simulink model "simIC"  (R2023b)
settings: Solver=VariableStepAuto  StartTime=0.0  StopTime=100.0  RelTol=1e-3
values from neighbouring files (symbols this model uses):
  beta = .1    (= 0.1)    [runIC.m]
  D_d = eye(6)*3    [runIC.m]
  dragcoeff = [C_d_1, C_d_4, C_d_C, C_d_L, beta, gamma]    [runIC.m]
  G_d = eye(6)*0.5    [runIC.m]
  gamma = .1    (= 0.1)    [runIC.m]
  K_D = blkdiag(eye(3),eye(3),eye(9))*500    [runIC.m]
  K_DI = diag([0.5 0.5 0.5 0.1 0.1 0.1])*2    [runIC.m]
  K_II = diag([0.2 0.2 0.2 0.15 0.15 0.15]*20)    [runIC.m]
  K_P = blkdiag(eye(3),eye(3),eye(9)*30)    [runIC.m]
  K_SI = diag([1 1 1 0.2 0.2 0.2])*30    [runIC.m]
  Lambda = blkdiag(eye(3)*40,eye(3)*40,eye(9)*40)    [runIC.m]
  M_d = eye(6)*4    [runIC.m]
  pos_init = [-0.02 (2*0.77*cos(pi/4)+1) 0]    [runIC.m]
  quat_init = eul2quat([0 0 pi],'XYZ')    [runIC.m]
  theta_init = [0 pi/4 0 pi/4 pi/4 0 pi/4 0 0]    [runIC.m]
  x_init = [pos_init quat_init theta_init zeta_init]'    [runIC.m]
undefined symbols (not defined in the file or in its folder): dt_MPC, pp, snake
libraries: dspindex x4, cstblocks x3
settings Model: Creator=sarava  LastModifiedBy=asker
settings SolverCC: AlgebraicLoopSolver=TrustRegion
settings DataIOCC: ReturnWorkspaceOutputs=off
settings DebuggingCC: UnconnectedInputMsg=warning  UnconnectedOutputMsg=warning  UnconnectedLineMsg=warning  ArithmeticOperatorsInVariantConditions=warning
settings ModelReferenceCC: EnableRefExpFcnMdlSchedulingChecks=on
settings SFSimCC: SimUseLocalCustomCode=off  CustomCodeUndefinedFunction=UseInterfaceOnly
settings RTWCC: RTWUseLocalCustomCode=off

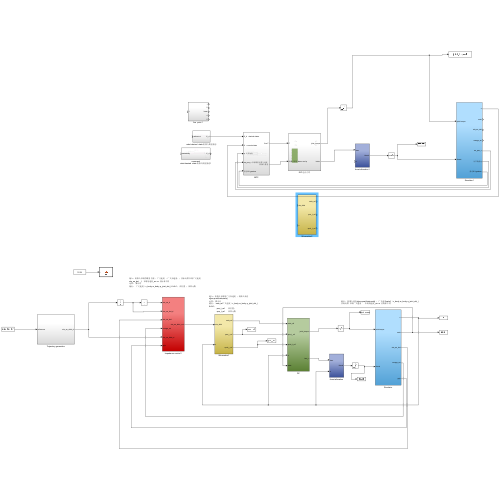
[thumbnail: Simulink's stored preview of the top-level diagram]
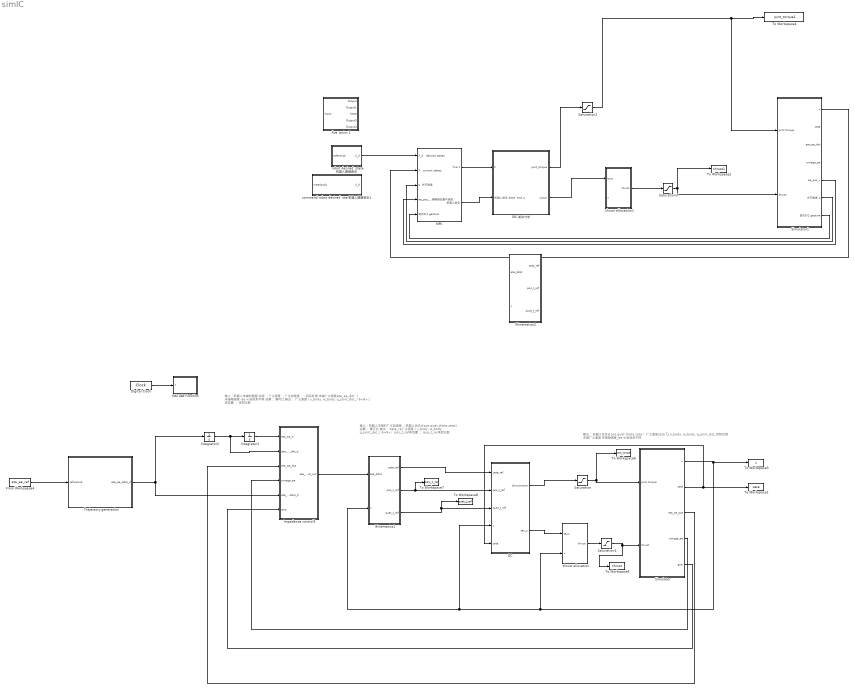
== system simIC ==
  note: 输入：机器人末端的广义加速度  ；机器人状态x[pos,quat,theta,zeta]
      | 运算： 雅可比
      | 输出：  zeta_ref广义速度（v_body, w_body, q_joint_dot_) 6+8+1；
      | 		pos_t_ref  	体位置 ；
      | 		qua_t_ref 	体四元数
  note: 输入：机器人末端的期望 位姿 ，广义速度  ，广义加速度，；实际反馈 末端广义速度eta_ee_dot   _I   末端角速度_ee  w  坐标系不同
      | 运算： 雅可比
      | 输出：  广义速度（v_body, w_body, q_joint_dot_) 6+8+1； 体位置 ； 体四元数
  note: 输出： 机器人状态x[pos,quat,theta,zeta]  ； 广义速度zeta ζ（v_body, w_body, q_joint_dot_)
      | 实际反馈  末端广义速度       末端角速度_ee  w  坐标系不同
  DC : Subsystem
  Digital Clock : DigitalClock
  From Workspace4 : FromWorkspace  VariableName=eta_ee_ref
  IDC 逆动力学 : Subsystem
  IKinematics1 : Subsystem
  IKinematics2 : Subsystem
  Impedance control1 : Subsystem
  Integrator1 : Integrator
  Integrator2 : Integrator
  MATLAB Function : MATLAB Function  TreatAsAtomicUnit=on
  MPC : Subsystem
  Saturation : Saturate  UpperLimit=8  LowerLimit=-2  ZeroCross=off
  Saturation1 : Saturate  UpperLimit=5  LowerLimit=-5  ZeroCross=off
  Saturation2 : Saturate  UpperLimit=8  LowerLimit=-2  ZeroCross=off
  Saturation3 : Saturate  UpperLimit=5  LowerLimit=-5  ZeroCross=off
  Simulator : Subsystem
  Simulator1 : Subsystem
  To Workspace1 : ToWorkspace  VariableName=zeta  SaveFormat=Timeseries  SampleTime=-1
  To Workspace2 : ToWorkspace  VariableName=thrust1  SaveFormat=Timeseries  SampleTime=-1
  To Workspace3 : ToWorkspace  VariableName=x  SaveFormat=Timeseries  SampleTime=-1
  To Workspace4 : ToWorkspace  VariableName=joint_torque1  SaveFormat=Timeseries  SampleTime=-1
  To Workspace5 : ToWorkspace  VariableName=thrust  SaveFormat=Timeseries  SampleTime=-1
  To Workspace6 : ToWorkspace  VariableName=joint_torque  SaveFormat=Timeseries  SampleTime=-1
  To Workspace7 : ToWorkspace  VariableName=pos_t_ref  SaveFormat=Timeseries  SampleTime=-1
  To Workspace8 : ToWorkspace  VariableName=quat_t_ref  SaveFormat=Timeseries  SampleTime=-1
  "Trajectory generation " : Subsystem
  command robot desired  state 机器人期望姿态1 : Subsystem
  five  point 1 : Subsystem
  robot desired  state 机器人期望姿态 : Subsystem
  thrust allocation : Subsystem
  thrust allocation1 : Subsystem
  wires:
  Digital Clock/1 -> MATLAB Function/1(t)
  thrust allocation/1(thrust) -> Saturation1/1
  Simulator/2(zeta) -> To Workspace1/1, DC/5("zeta ")
  Simulator/1(x) -> To Workspace3/1, DC/4(x), IKinematics1/2(x), thrust allocation/2("x ")
  IKinematics1/2(pos_t_ref) -> DC/2(pos_t_ref), To Workspace7/1
  IKinematics1/1(zeta_ref) -> DC/1(zeta_ref)
  IKinematics1/3(quat_t_ref) -> To Workspace8/1, DC/3(quat_t_ref)
  From Workspace4/1 -> "Trajectory generation "/1(reference)
  Integrator2/1 -> Impedance control1/2(eta_ee_dot_d), Integrator1/1
  "Trajectory generation "/1(eta_ee_ddot_d) -> Integrator2/1, Impedance control1/5(eta_ee_ddot_d)
  Simulator/3(eta_ee_dot) -> Impedance control1/3(eta_ee_dot)
  Simulator/4(omega_ee) -> Impedance control1/4(omega_ee)
  Integrator1/1 -> Impedance control1/1(eta_ee_d)
  Impedance control1/1(eta_ee_ddot_out) -> IKinematics1/1(eta_ddot)
  Simulator/5(grip) -> Impedance control1/6(grip)
  Saturation/1 -> To Workspace6/1, Simulator/1(joint torque)
  Saturation1/1 -> To Workspace5/1, Simulator/2(thrust)
  DC/1(joint_torque) -> Saturation/1
  DC/2(tau_c) -> thrust allocation/1("tauc ")
  Saturation2/1 -> To Workspace4/1, Simulator1/1(joint torque)
  IDC 逆动力学/1(joint_torque) -> Saturation2/1
  Saturation3/1 -> To Workspace2/1, Simulator1/2(thrust)
  thrust allocation1/1(thrust) -> Saturation3/1
  IDC 逆动力学/2("turtor ") -> thrust allocation1/1("tauc ")
  MPC/1(five F) -> IDC 逆动力学/1(F)
  MPC/2("机器人姿态 ") -> IDC 逆动力学/2(机器人姿态 base  and q)
  Simulator1/1(x) -> MPC/2(X   current states)
  Simulator1/6(关节角度 q) -> MPC/3(q  关节角度)
  Simulator1/5(ee_pos_v) -> MPC/4(ee_pos_v 末端期望位置与速度)
  robot desired  state 机器人期望姿态/1(X_d) -> MPC/1(X_d   desired states)
  Simulator1/7(姿态0/1 gesture) -> MPC/5(姿态0/1 gesture)

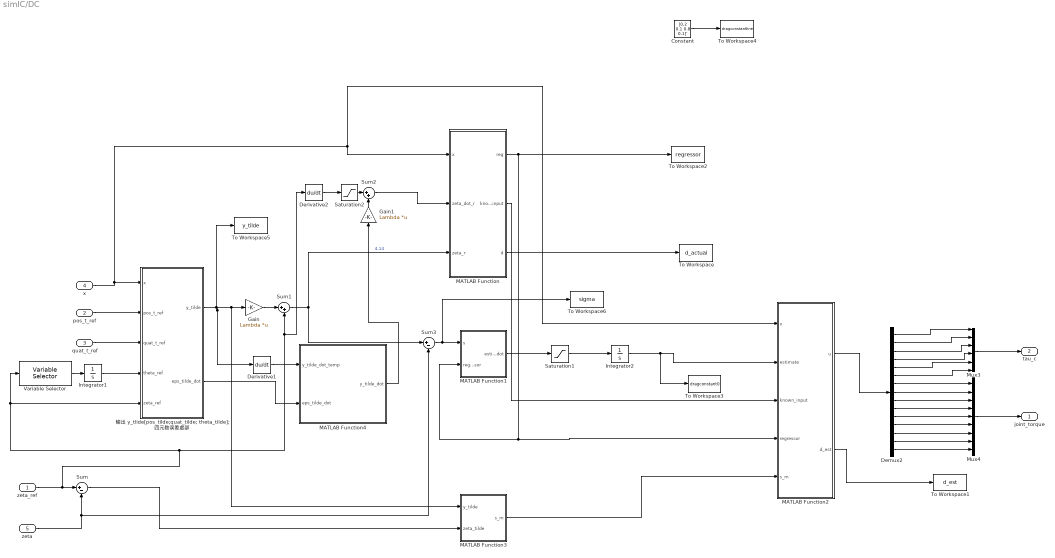
== system simIC/DC ==
  zeta_ref : Inport
  pos_t_ref : Inport  Port=2
  quat_t_ref : Inport  Port=3
  x : Inport  Port=4
  "zeta " : Inport  Port=5
  Constant : Constant  Value=[0.2 0.1 0.8 0.1]'
  Demux2 : Demux  Outputs=15
  Derivative1 : Derivative  CoefficientInTFapproximation=10
  Derivative2 : Derivative  CoefficientInTFapproximation=10
  Gain : Gain  Gain=Lambda  Multiplication=Matrix(K*u) (u vector)
  Gain1 : Gain  Gain=Lambda  Multiplication=Matrix(K*u) (u vector)
  Integrator1 : Integrator  InitialCondition=theta_init
  Integrator2 : Integrator  InitialCondition=[0 0 0 0]'
  MATLAB Function : MATLAB Function  TreatAsAtomicUnit=on
  MATLAB Function1 : MATLAB Function  TreatAsAtomicUnit=on
  MATLAB Function2 : MATLAB Function  TreatAsAtomicUnit=on
  MATLAB Function3 : MATLAB Function  TreatAsAtomicUnit=on
  MATLAB Function4 : MATLAB Function  TreatAsAtomicUnit=on
  Mux3 : Mux  Inputs=6
  Mux4 : Mux  Inputs=9
  Saturation1 : Saturate  UpperLimit=50  LowerLimit=-50  ZeroCross=off
  Saturation2 : Saturate  UpperLimit=20  LowerLimit=-20  ZeroCross=off
  Sum : Sum  Inputs=|+-
  Sum1 : Sum  Inputs=|++
  Sum2 : Sum  Inputs=|++
  Sum3 : Sum  Inputs=|+-
  To Workspace : ToWorkspace  VariableName=d_actual  SaveFormat=Timeseries  SampleTime=-1
  To Workspace1 : ToWorkspace  VariableName=d_est  SaveFormat=Timeseries  SampleTime=-1
  To Workspace2 : ToWorkspace  VariableName=regressor  SaveFormat=Timeseries  SampleTime=-1
  To Workspace3 : ToWorkspace  VariableName=dragconstant0  SaveFormat=Timeseries  SampleTime=-1
  To Workspace4 : ToWorkspace  VariableName=dragconstantline  SaveFormat=Timeseries  SampleTime=-1
  To Workspace5 : ToWorkspace  VariableName=y_tilde  SaveFormat=Timeseries  SampleTime=-1
  To Workspace6 : ToWorkspace  VariableName=sigma  SaveFormat=Timeseries  SampleTime=-1
  Variable Selector : dspindex/Variable Selector  NumInputs=1  rowsOrCols=Rows  IdxMode=Fixed  Elements=7:15  ZerOneIdxMode=One-based  errmode=Clip Index  FillMode=on  FillValues=0
  输出 y_tlide[pos_tilde;quat_tilde; theta_tilde]; 四元数误差虚部 : MATLAB Function  TreatAsAtomicUnit=on
  joint_torque : Outport  VectorParamsAs1DForOutWhenUnconnected=off
  tau_c : Outport  Port=2  VectorParamsAs1DForOutWhenUnconnected=off
  wires:
  x/1 -> MATLAB Function/1(x), MATLAB Function2/1(x), 输出 y_tlide[pos_tilde;quat_tilde; theta_tilde]; 四元数误差虚部/1(x)
  pos_t_ref/1 -> 输出 y_tlide[pos_tilde;quat_tilde; theta_tilde]; 四元数误差虚部/2(pos_t_ref)
  quat_t_ref/1 -> 输出 y_tlide[pos_tilde;quat_tilde; theta_tilde]; 四元数误差虚部/3(quat_t_ref)
  zeta_ref/1 -> Derivative2/1, Sum1/2, Variable Selector/1, 输出 y_tlide[pos_tilde;quat_tilde; theta_tilde]; 四元数误差虚部/5(zeta_ref), Sum/1
  "zeta "/1 -> Sum3/2, Sum/2
  Integrator1/1 -> 输出 y_tlide[pos_tilde;quat_tilde; theta_tilde]; 四元数误差虚部/4(theta_ref)
  输出 y_tlide[pos_tilde;quat_tilde; theta_tilde]; 四元数误差虚部/1(y_tilde) -> MATLAB Function3/1(y_tilde), Gain/1, Derivative1/1, To Workspace5/1
  Gain/1 -> Sum1/1
  Sum1/1 -> Sum3/1, MATLAB Function/3(zeta_r)  "4.14"
  Saturation1/1 -> Integrator2/1
  MATLAB Function1/1(estimate_dot) -> Saturation1/1
  MATLAB Function3/1(s_m) -> MATLAB Function2/5(s_m)
  MATLAB Function2/1(u) -> Demux2/1
  Demux2/14 -> Mux4/8
  Demux2/4 -> Mux3/4
  Demux2/5 -> Mux3/5
  Demux2/12 -> Mux4/6
  Demux2/2 -> Mux3/2
  Demux2/9 -> Mux4/3
  Demux2/3 -> Mux3/3
  Demux2/13 -> Mux4/7
  Demux2/8 -> Mux4/2
  Demux2/6 -> Mux3/6
  Demux2/10 -> Mux4/4
  Demux2/7 -> Mux4/1
  Demux2/11 -> Mux4/5
  Demux2/1 -> Mux3/1
  Mux4/1 -> joint_torque/1
  Mux3/1 -> tau_c/1
  Variable Selector/1 -> Integrator1/1
  Integrator2/1 -> To Workspace3/1, MATLAB Function2/2(estimate)
  MATLAB Function/2(known_input) -> MATLAB Function2/3(known_input)
  MATLAB Function/1(reg) -> To Workspace2/1, MATLAB Function1/2(regressor), MATLAB Function2/4(regressor)
  输出 y_tlide[pos_tilde;quat_tilde; theta_tilde]; 四元数误差虚部/2(eps_tilde_dot) -> MATLAB Function4/2(eps_tilde_dot)
  Derivative1/1 -> MATLAB Function4/1(y_tilde_dot_temp)
  MATLAB Function4/1(y_tilde_dot) -> Gain1/1
  Derivative2/1 -> Saturation2/1
  Saturation2/1 -> Sum2/1
  Gain1/1 -> Sum2/2
  Sum3/1 -> To Workspace6/1, MATLAB Function1/1(s)
  Sum2/1 -> MATLAB Function/2(zeta_dot_r)
  Sum/1 -> MATLAB Function3/2(zeta_tilde)
  MATLAB Function/3(d) -> To Workspace/1
  MATLAB Function2/2(d_est) -> To Workspace1/1
  Constant/1 -> To Workspace4/1
  Demux2/15 -> Mux4/9

== system simIC/IDC 逆动力学 ==
  F : Inport
  机器人姿态 base  and q : Inport  Port=2
  DC : Subsystem
  joint_torque : Outport
  "turtor " : Outport  Port=2

== system simIC/IKinematics1 ==
  eta_ddot : Inport
  x : Inport  Port=2
  Integrator3 : Integrator
  Integrator5 : Integrator  InitialCondition=[pos_init quat_init]'
  MATLAB Function1 : MATLAB Function  TreatAsAtomicUnit=on
  zeta_ref : Outport  VectorParamsAs1DForOutWhenUnconnected=off
  pos_t_ref : Outport  Port=2  VectorParamsAs1DForOutWhenUnconnected=off
  quat_t_ref : Outport  Port=3  VectorParamsAs1DForOutWhenUnconnected=off
  wires:
  x/1 -> MATLAB Function1/2(x)
  MATLAB Function1/1(zeta_ref) -> zeta_ref/1
  MATLAB Function1/2(pos_t_ref) -> pos_t_ref/1
  eta_ddot/1 -> Integrator3/1
  Integrator3/1 -> MATLAB Function1/1(eta_ee_d_dot)
  MATLAB Function1/3(eta_t_dot_quat_ref) -> Integrator5/1
  Integrator5/1 -> MATLAB Function1/3(eta_t_ref)
  MATLAB Function1/4(quatt_ref) -> quat_t_ref/1

== system simIC/IKinematics2 ==
  eta_ddot : Inport
  x : Inport  Port=2
  Integrator3 : Integrator
  Integrator5 : Integrator  InitialCondition=[pos_init quat_init]'
  MATLAB Function1 : MATLAB Function  TreatAsAtomicUnit=on
  zeta_ref : Outport  VectorParamsAs1DForOutWhenUnconnected=off
  pos_t_ref : Outport  Port=2  VectorParamsAs1DForOutWhenUnconnected=off
  quat_t_ref : Outport  Port=3  VectorParamsAs1DForOutWhenUnconnected=off
  wires:
  x/1 -> MATLAB Function1/3(x)
  MATLAB Function1/1(zeta_ref) -> zeta_ref/1
  MATLAB Function1/2(pos_t_ref) -> pos_t_ref/1
  eta_ddot/1 -> Integrator3/1
  Integrator3/1 -> MATLAB Function1/1(eta_zuo_d_dot)
  MATLAB Function1/3(eta_t_dot_quat_ref) -> Integrator5/1
  Integrator5/1 -> MATLAB Function1/4(eta_t_ref)
  MATLAB Function1/4(quatt_ref) -> quat_t_ref/1

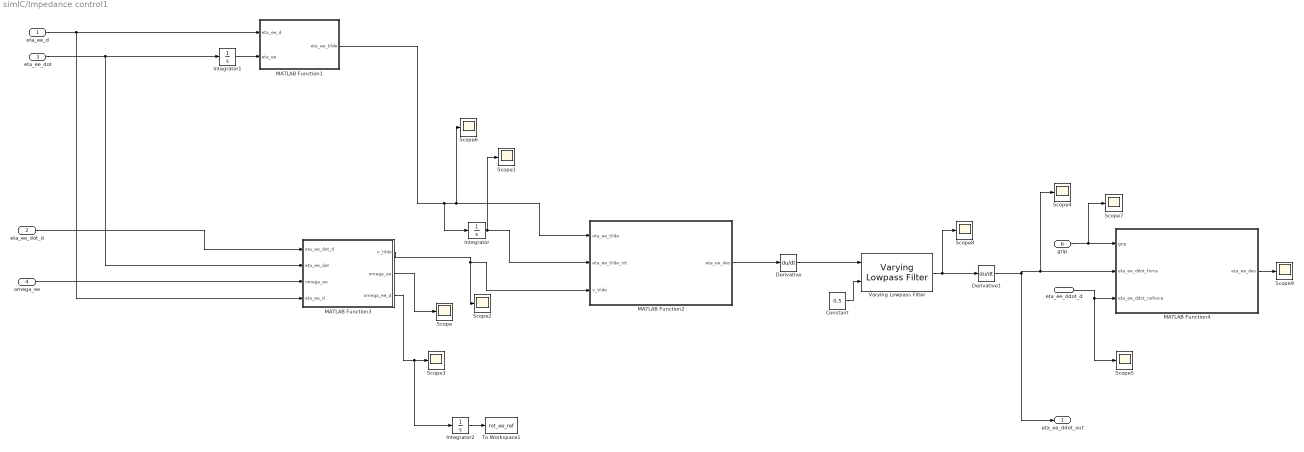
== system simIC/Impedance control1 ==
  eta_ee_d : Inport
  eta_ee_dot_d : Inport  Port=2
  eta_ee_dot : Inport  Port=3
  omega_ee : Inport  Port=4
  eta_ee_ddot_d : Inport  Port=5
  grip : Inport  Port=6
  Constant : Constant  Value=0.5
  Derivative : Derivative
  Derivative1 : Derivative
  Integrator : Integrator
  Integrator1 : Integrator
  Integrator2 : Integrator
  MATLAB Function1 : MATLAB Function  TreatAsAtomicUnit=on
  MATLAB Function2 : MATLAB Function  TreatAsAtomicUnit=on
  MATLAB Function3 : MATLAB Function  TreatAsAtomicUnit=on
  MATLAB Function4 : MATLAB Function  TreatAsAtomicUnit=on
  Scope{,1..9} (10 alike) : Scope
  To Workspace1 : ToWorkspace  VariableName=rot_ee_ref  SaveFormat=Timeseries  SampleTime=-1
  Varying Lowpass Filter : cstblocks/Linear Parameter Varying/Varying Lowpass Filter  N=1
  eta_ee_ddot_out : Outport  VectorParamsAs1DForOutWhenUnconnected=off
  wires:
  eta_ee_d/1 -> MATLAB Function3/4(eta_ee_d), MATLAB Function1/1(eta_ee_d)
  eta_ee_dot_d/1 -> MATLAB Function3/1(eta_ee_dot_d)
  eta_ee_dot/1 -> Integrator1/1, MATLAB Function3/2(eta_ee_dot)
  omega_ee/1 -> MATLAB Function3/3("omega_ee ")
  MATLAB Function3/1(v_tilde) -> MATLAB Function2/3(v_tilde), Scope2/1
  MATLAB Function1/1(eta_ee_tilde) -> Integrator/1, Scope6/1, MATLAB Function2/1(eta_ee_tilde)
  Integrator/1 -> Scope1/1, MATLAB Function2/2(eta_ee_tilde_int)
  MATLAB Function3/2(omega_ee) -> Scope/1
  MATLAB Function2/1(eta_ee_des) -> Derivative/1
  Integrator1/1 -> MATLAB Function1/2(eta_ee)
  MATLAB Function3/3(omega_ee_d) -> Integrator2/1, Scope3/1
  Constant/1 -> Varying Lowpass Filter/2
  Derivative/1 -> Varying Lowpass Filter/1
  Varying Lowpass Filter/1 -> Derivative1/1, Scope8/1
  Integrator2/1 -> To Workspace1/1
  grip/1 -> Scope7/1, MATLAB Function4/1(grip)
  Derivative1/1 -> eta_ee_ddot_out/1, Scope4/1, MATLAB Function4/2(eta_ee_ddot_force)
  eta_ee_ddot_d/1 -> Scope5/1, MATLAB Function4/3(eta_ee_ddot_noforce)
  MATLAB Function4/1(eta_ee_des) -> Scope9/1

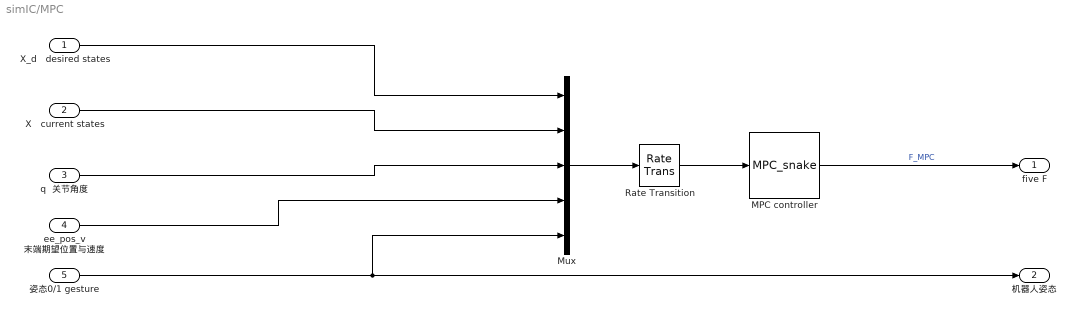
== system simIC/MPC ==
  X_d   desired states : Inport
  X   current states : Inport  Port=2
  q  关节角度 : Inport  Port=3
  ee_pos_v 末端期望位置与速度 : Inport  Port=4
  姿态0/1 gesture : Inport  Port=5
  MPC controller : MATLABFcn  MATLABFcn=MPC_snake  OutputDimensions=[12 1]  Output1D=off
  Mux : Mux  Inputs=5
  Rate Transition : RateTransition  OutPortSampleTime=dt_MPC/5
  five F : Outport
  "机器人姿态 " : Outport  Port=2
  wires:
  Mux/1 -> Rate Transition/1
  X_d   desired states/1 -> Mux/1
  Rate Transition/1 -> MPC controller/1
  X   current states/1 -> Mux/2
  q  关节角度/1 -> Mux/3
  ee_pos_v 末端期望位置与速度/1 -> Mux/4
  姿态0/1 gesture/1 -> Mux/5, "机器人姿态 "/1
  MPC controller/1 -> five F/1  "F_MPC"

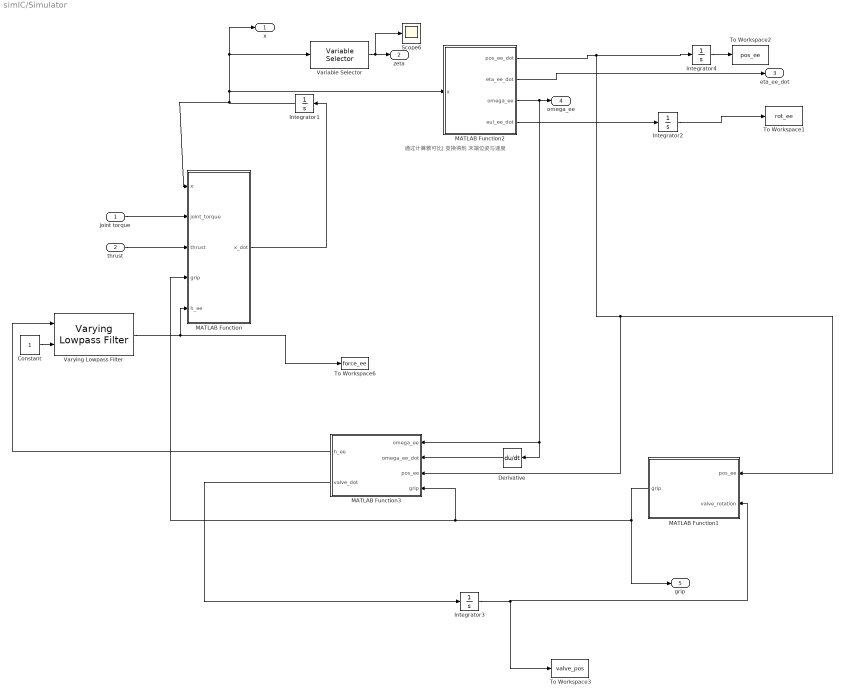
== system simIC/Simulator ==
  note: 通过计算雅可比J 变换得到 末端位姿与速度
  joint torque : Inport
  thrust : Inport  Port=2
  Constant : Constant
  Derivative : Derivative
  Integrator1 : Integrator  InitialCondition=x_init
  Integrator2 : Integrator
  Integrator3 : Integrator
  Integrator4 : Integrator
  MATLAB Function : MATLAB Function  TreatAsAtomicUnit=on
  MATLAB Function1 : MATLAB Function  TreatAsAtomicUnit=on
  MATLAB Function2 : MATLAB Function  TreatAsAtomicUnit=on
  MATLAB Function3 : MATLAB Function  TreatAsAtomicUnit=on
  Scope6 : Scope
  To Workspace1 : ToWorkspace  VariableName=rot_ee  SaveFormat=Timeseries  SampleTime=-1
  To Workspace2 : ToWorkspace  VariableName=pos_ee  SaveFormat=Timeseries  SampleTime=-1
  To Workspace3 : ToWorkspace  VariableName=valve_pos  SaveFormat=Timeseries  SampleTime=-1
  To Workspace6 : ToWorkspace  VariableName=force_ee  SaveFormat=Timeseries  SampleTime=-1
  Variable Selector : dspindex/Variable Selector  NumInputs=1  rowsOrCols=Rows  IdxMode=Fixed  Elements=17:31  ZerOneIdxMode=One-based  errmode=Clip Index  FillMode=on  FillValues=0
  Varying Lowpass Filter : cstblocks/Linear Parameter Varying/Varying Lowpass Filter  N=1
  x : Outport  VectorParamsAs1DForOutWhenUnconnected=off
  zeta : Outport  Port=2  VectorParamsAs1DForOutWhenUnconnected=off
  eta_ee_dot : Outport  Port=3  VectorParamsAs1DForOutWhenUnconnected=off
  omega_ee : Outport  Port=4  VectorParamsAs1DForOutWhenUnconnected=off
  grip : Outport  Port=5  VectorParamsAs1DForOutWhenUnconnected=off
  wires:
  joint torque/1 -> MATLAB Function/2(joint_torque)
  thrust/1 -> MATLAB Function/3(thrust)
  Variable Selector/1 -> Scope6/1, zeta/1
  MATLAB Function2/1(pos_ee_dot) -> Integrator4/1, MATLAB Function3/3(pos_ee), MATLAB Function1/1(pos_ee)
  MATLAB Function/1(x_dot) -> Integrator1/1
  Integrator1/1 -> Variable Selector/1, x/1, MATLAB Function2/1(x), MATLAB Function/1(x)
  MATLAB Function2/2(eta_ee_dot) -> eta_ee_dot/1
  MATLAB Function2/3(omega_ee) -> Derivative/1, MATLAB Function3/1(omega_ee), omega_ee/1
  Integrator2/1 -> To Workspace1/1
  MATLAB Function3/1(h_ee) -> Varying Lowpass Filter/1
  MATLAB Function1/1(grip) -> MATLAB Function3/4(grip), MATLAB Function/4(grip), grip/1
  MATLAB Function3/2(valve_dot) -> Integrator3/1
  Integrator3/1 -> MATLAB Function1/2(valve_rotation), To Workspace3/1
  Derivative/1 -> MATLAB Function3/2(omega_ee_dot)
  Varying Lowpass Filter/1 -> MATLAB Function/5(h_ee), To Workspace6/1
  Constant/1 -> Varying Lowpass Filter/2
  Integrator4/1 -> To Workspace2/1
  MATLAB Function2/4(eul_ee_dot) -> Integrator2/1

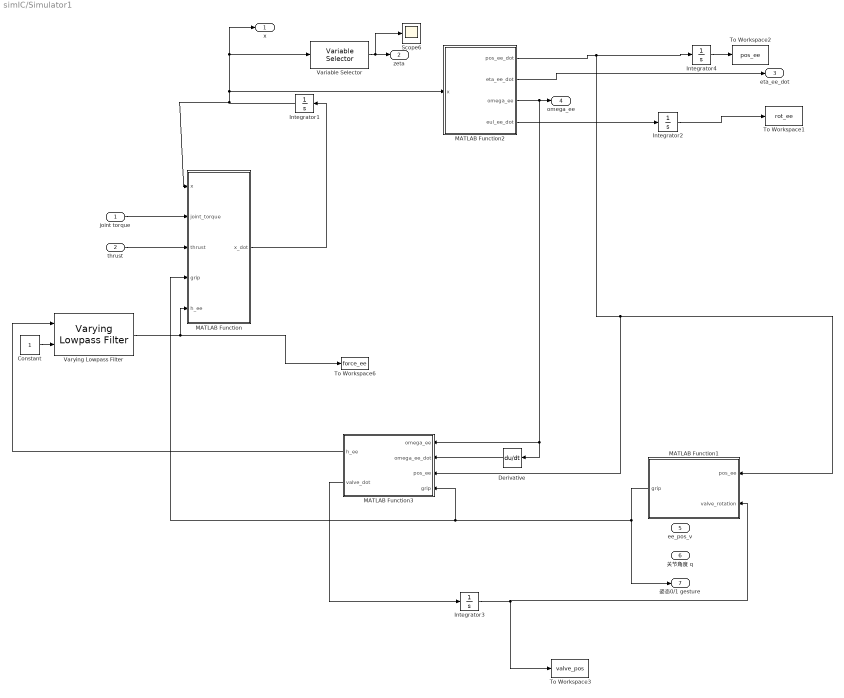
== system simIC/Simulator1 ==
  joint torque : Inport
  thrust : Inport  Port=2
  Constant : Constant
  Derivative : Derivative
  Integrator1 : Integrator  InitialCondition=x_init
  Integrator2 : Integrator
  Integrator3 : Integrator
  Integrator4 : Integrator
  MATLAB Function : MATLAB Function  TreatAsAtomicUnit=on
  MATLAB Function1 : MATLAB Function  TreatAsAtomicUnit=on
  MATLAB Function2 : MATLAB Function  TreatAsAtomicUnit=on
  MATLAB Function3 : MATLAB Function  TreatAsAtomicUnit=on
  Scope6 : Scope
  To Workspace1 : ToWorkspace  VariableName=rot_ee  SaveFormat=Timeseries  SampleTime=-1
  To Workspace2 : ToWorkspace  VariableName=pos_ee  SaveFormat=Timeseries  SampleTime=-1
  To Workspace3 : ToWorkspace  VariableName=valve_pos  SaveFormat=Timeseries  SampleTime=-1
  To Workspace6 : ToWorkspace  VariableName=force_ee  SaveFormat=Timeseries  SampleTime=-1
  Variable Selector : dspindex/Variable Selector  NumInputs=1  rowsOrCols=Rows  IdxMode=Fixed  Elements=17:31  ZerOneIdxMode=One-based  errmode=Clip Index  FillMode=on  FillValues=0
  Varying Lowpass Filter : cstblocks/Linear Parameter Varying/Varying Lowpass Filter  N=1
  x : Outport  VectorParamsAs1DForOutWhenUnconnected=off
  zeta : Outport  Port=2  VectorParamsAs1DForOutWhenUnconnected=off
  eta_ee_dot : Outport  Port=3  VectorParamsAs1DForOutWhenUnconnected=off
  omega_ee : Outport  Port=4  VectorParamsAs1DForOutWhenUnconnected=off
  ee_pos_v : Outport  Port=5
  关节角度 q : Outport  Port=6
  姿态0/1 gesture : Outport  Port=7  VectorParamsAs1DForOutWhenUnconnected=off
  wires:
  joint torque/1 -> MATLAB Function/2(joint_torque)
  thrust/1 -> MATLAB Function/3(thrust)
  Variable Selector/1 -> Scope6/1, zeta/1
  MATLAB Function2/1(pos_ee_dot) -> Integrator4/1, MATLAB Function3/3(pos_ee), MATLAB Function1/1(pos_ee)
  MATLAB Function/1(x_dot) -> Integrator1/1
  Integrator1/1 -> Variable Selector/1, x/1, MATLAB Function2/1(x), MATLAB Function/1(x)
  MATLAB Function2/2(eta_ee_dot) -> eta_ee_dot/1
  MATLAB Function2/3(omega_ee) -> Derivative/1, MATLAB Function3/1(omega_ee), omega_ee/1
  Integrator2/1 -> To Workspace1/1
  MATLAB Function3/1(h_ee) -> Varying Lowpass Filter/1
  MATLAB Function1/1(grip) -> MATLAB Function3/4(grip), MATLAB Function/4(grip), 姿态0/1 gesture/1
  MATLAB Function3/2(valve_dot) -> Integrator3/1
  Integrator3/1 -> MATLAB Function1/2(valve_rotation), To Workspace3/1
  Derivative/1 -> MATLAB Function3/2(omega_ee_dot)
  Varying Lowpass Filter/1 -> MATLAB Function/5(h_ee), To Workspace6/1
  Constant/1 -> Varying Lowpass Filter/2
  Integrator4/1 -> To Workspace2/1
  MATLAB Function2/4(eul_ee_dot) -> Integrator2/1

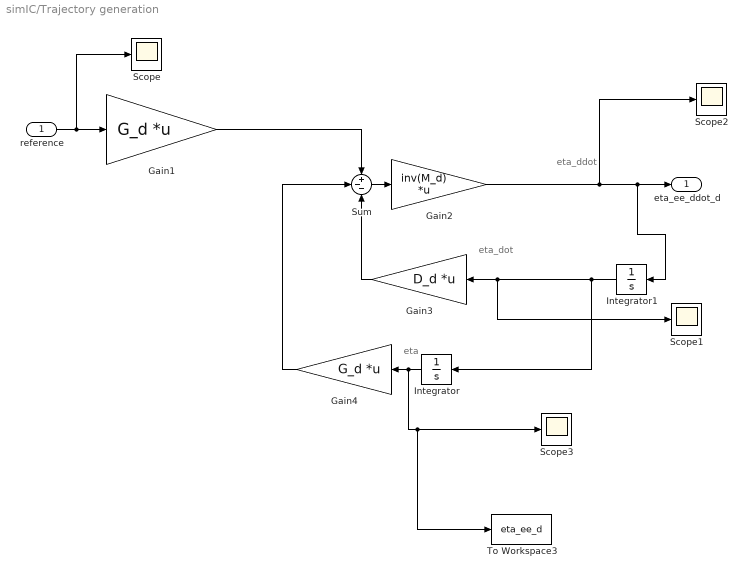
== system simIC/Trajectory generation  ==
  note: eta_dot
  note: eta
  note: eta_ddot
  reference : Inport
  Gain1 : Gain  Gain=G_d  Multiplication=Matrix(K*u) (u vector)
  Gain2 : Gain  Gain=inv(M_d)  Multiplication=Matrix(K*u) (u vector)
  Gain3 : Gain  Gain=D_d  Multiplication=Matrix(K*u) (u vector)
  Gain4 : Gain  Gain=G_d  Multiplication=Matrix(K*u) (u vector)
  Integrator : Integrator
  Integrator1 : Integrator
  Scope{,1..3} (4 alike) : Scope
  Sum : Sum  Inputs=+--
  To Workspace3 : ToWorkspace  VariableName=eta_ee_d  SaveFormat=Timeseries  SampleTime=-1
  eta_ee_ddot_d : Outport  VectorParamsAs1DForOutWhenUnconnected=off
  wires:
  Gain2/1 -> Scope2/1, eta_ee_ddot_d/1, Integrator1/1
  Gain1/1 -> Sum/1
  Sum/1 -> Gain2/1
  reference/1 -> Scope/1, Gain1/1
  Integrator1/1 -> Integrator/1, Scope1/1, Gain3/1
  Integrator/1 -> To Workspace3/1, Scope3/1, Gain4/1
  Gain3/1 -> Sum/3
  Gain4/1 -> Sum/2

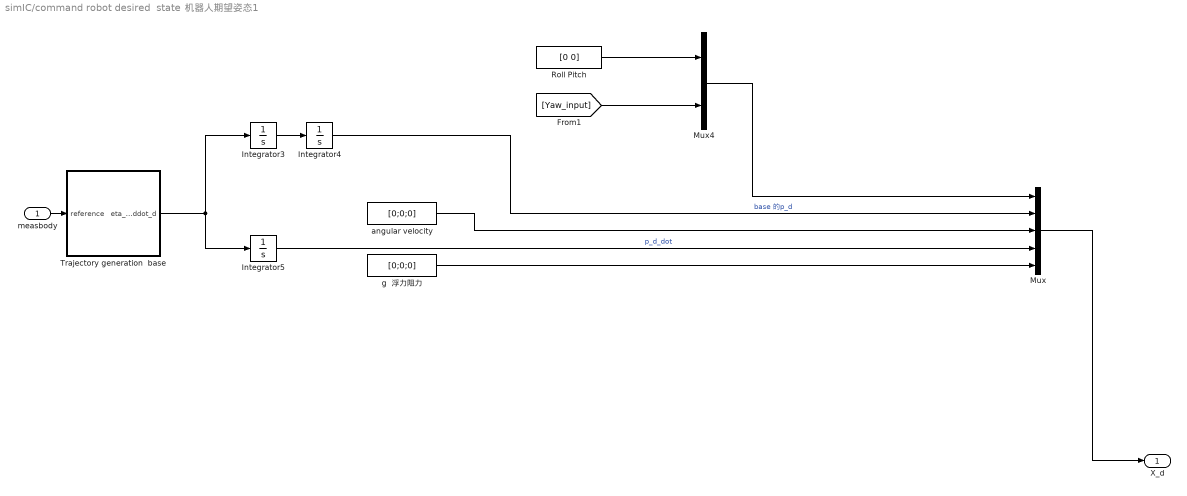
== system simIC/command robot desired  state 机器人期望姿态1 ==
  measbody : Inport
  Integrator3 : Integrator
  Integrator4 : Integrator
  Integrator5 : Integrator
  Mux : Mux  Inputs=5
  Mux4 : Mux  Inputs=2
  Roll Pitch : Constant  Value=[0 0]
  Trajectory generation  base : Subsystem
  angular velocity : Constant  Value=[0;0;0]
  g  浮力阻力 : Constant  Value=[0;0;0]
  X_d : Outport
  wires:
  Mux/1 -> X_d/1
  Mux4/1 -> Mux/1
  Integrator3/1 -> Integrator4/1
  [Yaw_input] -> Mux4/2
  g  浮力阻力/1 -> Mux/5
  Integrator5/1 -> Mux/4  "p_d_dot"
  Trajectory generation  base/1(eta_ee_ddot_d) -> Integrator3/1, Integrator5/1
  Roll Pitch/1 -> Mux4/1
  angular velocity/1 -> Mux/3
  measbody/1 -> Trajectory generation  base/1(reference)
  Integrator4/1 -> Mux/2  "base 的p_d"

== system simIC/five  point 1 ==
  Input : Inport
  Output : Outport
  Output1 : Outport  Port=2
  base : Outport  Port=3
  Output3 : Outport  Port=4
  Output4 : Outport  Port=5
  wires:
  Input/1 -> base/1

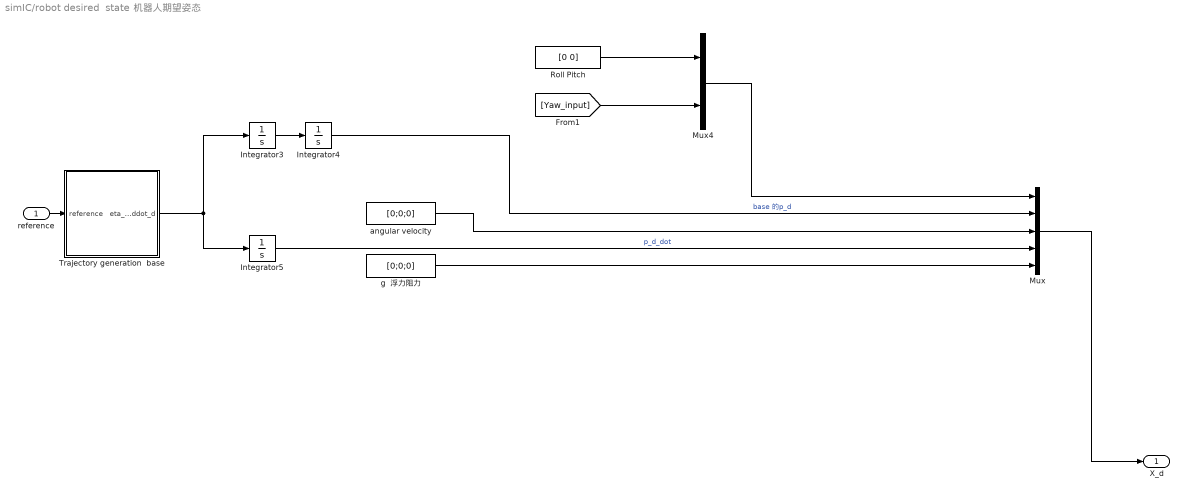
== system simIC/robot desired  state 机器人期望姿态 ==
  reference : Inport
  Integrator3 : Integrator
  Integrator4 : Integrator
  Integrator5 : Integrator
  Mux : Mux  Inputs=5
  Mux4 : Mux  Inputs=2
  Roll Pitch : Constant  Value=[0 0]
  Trajectory generation  base : Subsystem
  angular velocity : Constant  Value=[0;0;0]
  g  浮力阻力 : Constant  Value=[0;0;0]
  X_d : Outport
  wires:
  Mux/1 -> X_d/1
  Mux4/1 -> Mux/1
  Integrator3/1 -> Integrator4/1
  [Yaw_input] -> Mux4/2
  g  浮力阻力/1 -> Mux/5
  Integrator5/1 -> Mux/4  "p_d_dot"
  Trajectory generation  base/1(eta_ee_ddot_d) -> Integrator3/1, Integrator5/1
  Roll Pitch/1 -> Mux4/1
  angular velocity/1 -> Mux/3
  reference/1 -> Trajectory generation  base/1(reference)
  Integrator4/1 -> Mux/2  "base 的p_d"

== system simIC/thrust allocation ==
  "tauc " : Inport
  "x " : Inport  Port=2
  MATLAB Function : MATLAB Function  TreatAsAtomicUnit=on
  Product : Product  Multiplication=Matrix(*)
  thrust : Outport  VectorParamsAs1DForOutWhenUnconnected=off
  wires:
  "x "/1 -> MATLAB Function/1(x)
  MATLAB Function/1(TCM) -> Product/1
  "tauc "/1 -> Product/2
  Product/1 -> thrust/1

== system simIC/thrust allocation1 ==
  "tauc " : Inport
  "x " : Inport  Port=2
  MATLAB Function : MATLAB Function  TreatAsAtomicUnit=on
  Product : Product  Multiplication=Matrix(*)
  thrust : Outport  VectorParamsAs1DForOutWhenUnconnected=off
  wires:
  "x "/1 -> MATLAB Function/1(x)
  MATLAB Function/1(TCM) -> Product/1
  "tauc "/1 -> Product/2
  Product/1 -> thrust/1

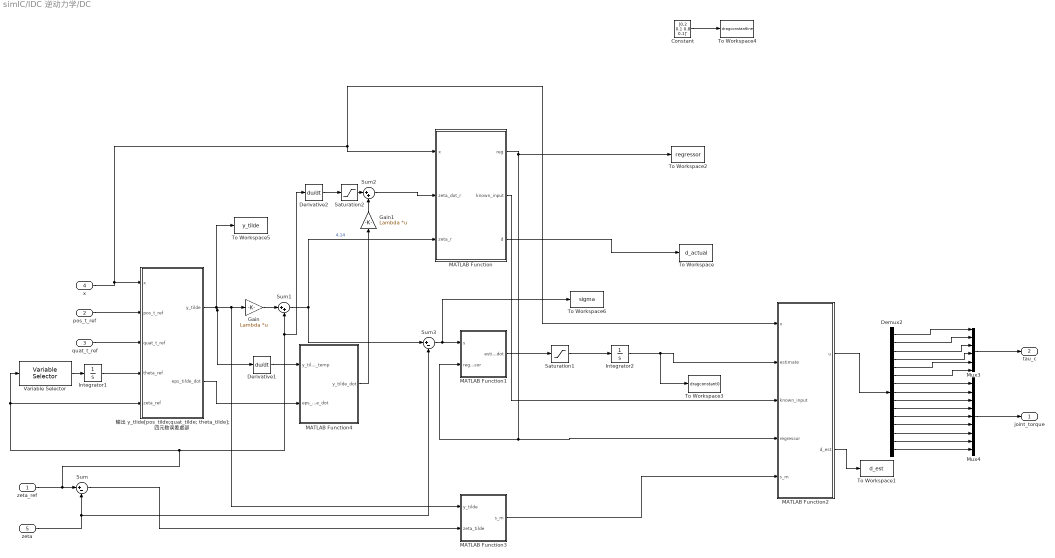
== system simIC/IDC 逆动力学/DC ==
  zeta_ref : Inport
  pos_t_ref : Inport  Port=2
  quat_t_ref : Inport  Port=3
  x : Inport  Port=4
  "zeta " : Inport  Port=5
  Constant : Constant  Value=[0.2 0.1 0.8 0.1]'
  Demux2 : Demux  Outputs=15
  Derivative1 : Derivative  CoefficientInTFapproximation=10
  Derivative2 : Derivative  CoefficientInTFapproximation=10
  Gain : Gain  Gain=Lambda  Multiplication=Matrix(K*u) (u vector)
  Gain1 : Gain  Gain=Lambda  Multiplication=Matrix(K*u) (u vector)
  Integrator1 : Integrator  InitialCondition=theta_init
  Integrator2 : Integrator  InitialCondition=[0 0 0 0]'
  MATLAB Function : MATLAB Function  TreatAsAtomicUnit=on
  MATLAB Function1 : MATLAB Function  TreatAsAtomicUnit=on
  MATLAB Function2 : MATLAB Function  TreatAsAtomicUnit=on
  MATLAB Function3 : MATLAB Function  TreatAsAtomicUnit=on
  MATLAB Function4 : MATLAB Function  TreatAsAtomicUnit=on
  Mux3 : Mux  Inputs=6
  Mux4 : Mux  Inputs=9
  Saturation1 : Saturate  UpperLimit=50  LowerLimit=-50  ZeroCross=off
  Saturation2 : Saturate  UpperLimit=20  LowerLimit=-20  ZeroCross=off
  Sum : Sum  Inputs=|+-
  Sum1 : Sum  Inputs=|++
  Sum2 : Sum  Inputs=|++
  Sum3 : Sum  Inputs=|+-
  To Workspace : ToWorkspace  VariableName=d_actual  SaveFormat=Timeseries  SampleTime=-1
  To Workspace1 : ToWorkspace  VariableName=d_est  SaveFormat=Timeseries  SampleTime=-1
  To Workspace2 : ToWorkspace  VariableName=regressor  SaveFormat=Timeseries  SampleTime=-1
  To Workspace3 : ToWorkspace  VariableName=dragconstant0  SaveFormat=Timeseries  SampleTime=-1
  To Workspace4 : ToWorkspace  VariableName=dragconstantline  SaveFormat=Timeseries  SampleTime=-1
  To Workspace5 : ToWorkspace  VariableName=y_tilde  SaveFormat=Timeseries  SampleTime=-1
  To Workspace6 : ToWorkspace  VariableName=sigma  SaveFormat=Timeseries  SampleTime=-1
  Variable Selector : dspindex/Variable Selector  NumInputs=1  rowsOrCols=Rows  IdxMode=Fixed  Elements=7:15  ZerOneIdxMode=One-based  errmode=Clip Index  FillMode=on  FillValues=0
  输出 y_tlide[pos_tilde;quat_tilde; theta_tilde]; 四元数误差虚部 : MATLAB Function  TreatAsAtomicUnit=on
  joint_torque : Outport  VectorParamsAs1DForOutWhenUnconnected=off
  tau_c : Outport  Port=2  VectorParamsAs1DForOutWhenUnconnected=off
  wires:
  x/1 -> MATLAB Function/1(x), MATLAB Function2/1(x), 输出 y_tlide[pos_tilde;quat_tilde; theta_tilde]; 四元数误差虚部/1(x)
  pos_t_ref/1 -> 输出 y_tlide[pos_tilde;quat_tilde; theta_tilde]; 四元数误差虚部/2(pos_t_ref)
  quat_t_ref/1 -> 输出 y_tlide[pos_tilde;quat_tilde; theta_tilde]; 四元数误差虚部/3(quat_t_ref)
  zeta_ref/1 -> Derivative2/1, Sum1/2, Variable Selector/1, 输出 y_tlide[pos_tilde;quat_tilde; theta_tilde]; 四元数误差虚部/5(zeta_ref), Sum/1
  "zeta "/1 -> Sum3/2, Sum/2
  Integrator1/1 -> 输出 y_tlide[pos_tilde;quat_tilde; theta_tilde]; 四元数误差虚部/4(theta_ref)
  输出 y_tlide[pos_tilde;quat_tilde; theta_tilde]; 四元数误差虚部/1(y_tilde) -> MATLAB Function3/1(y_tilde), Gain/1, Derivative1/1, To Workspace5/1
  Gain/1 -> Sum1/1
  Sum1/1 -> Sum3/1, MATLAB Function/3(zeta_r)  "4.14"
  Saturation1/1 -> Integrator2/1
  MATLAB Function1/1(estimate_dot) -> Saturation1/1
  MATLAB Function3/1(s_m) -> MATLAB Function2/5(s_m)
  MATLAB Function2/1(u) -> Demux2/1
  Demux2/14 -> Mux4/8
  Demux2/4 -> Mux3/4
  Demux2/5 -> Mux3/5
  Demux2/12 -> Mux4/6
  Demux2/2 -> Mux3/2
  Demux2/9 -> Mux4/3
  Demux2/3 -> Mux3/3
  Demux2/13 -> Mux4/7
  Demux2/8 -> Mux4/2
  Demux2/6 -> Mux3/6
  Demux2/10 -> Mux4/4
  Demux2/7 -> Mux4/1
  Demux2/11 -> Mux4/5
  Demux2/1 -> Mux3/1
  Mux4/1 -> joint_torque/1
  Mux3/1 -> tau_c/1
  Variable Selector/1 -> Integrator1/1
  Integrator2/1 -> To Workspace3/1, MATLAB Function2/2(estimate)
  MATLAB Function/2(known_input) -> MATLAB Function2/3(known_input)
  MATLAB Function/1(reg) -> To Workspace2/1, MATLAB Function1/2(regressor), MATLAB Function2/4(regressor)
  输出 y_tlide[pos_tilde;quat_tilde; theta_tilde]; 四元数误差虚部/2(eps_tilde_dot) -> MATLAB Function4/2(eps_tilde_dot)
  Derivative1/1 -> MATLAB Function4/1(y_tilde_dot_temp)
  MATLAB Function4/1(y_tilde_dot) -> Gain1/1
  Derivative2/1 -> Saturation2/1
  Saturation2/1 -> Sum2/1
  Gain1/1 -> Sum2/2
  Sum3/1 -> To Workspace6/1, MATLAB Function1/1(s)
  Sum2/1 -> MATLAB Function/2(zeta_dot_r)
  Sum/1 -> MATLAB Function3/2(zeta_tilde)
  MATLAB Function/3(d) -> To Workspace/1
  MATLAB Function2/2(d_est) -> To Workspace1/1
  Constant/1 -> To Workspace4/1
  Demux2/15 -> Mux4/9

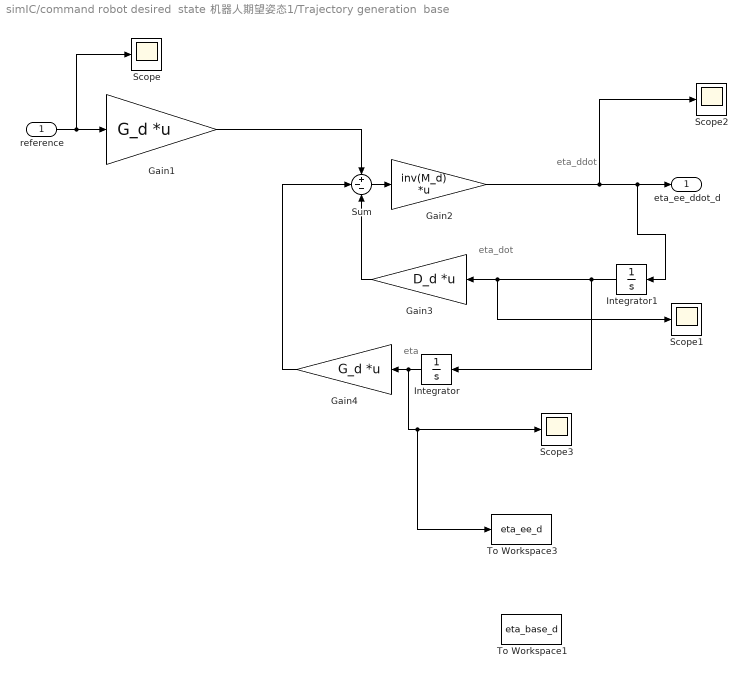
== system simIC/command robot desired  state 机器人期望姿态1/Trajectory generation  base ==
  note: eta_dot
  note: eta
  note: eta_ddot
  reference : Inport
  Gain1 : Gain  Gain=G_d  Multiplication=Matrix(K*u) (u vector)
  Gain2 : Gain  Gain=inv(M_d)  Multiplication=Matrix(K*u) (u vector)
  Gain3 : Gain  Gain=D_d  Multiplication=Matrix(K*u) (u vector)
  Gain4 : Gain  Gain=G_d  Multiplication=Matrix(K*u) (u vector)
  Integrator : Integrator
  Integrator1 : Integrator
  Scope{,1..3} (4 alike) : Scope
  Sum : Sum  Inputs=+--
  To Workspace1 : ToWorkspace  VariableName=eta_base_d  SaveFormat=Timeseries  SampleTime=-1
  To Workspace3 : ToWorkspace  VariableName=eta_ee_d  SaveFormat=Timeseries  SampleTime=-1
  eta_ee_ddot_d : Outport  VectorParamsAs1DForOutWhenUnconnected=off
  wires:
  Gain2/1 -> Scope2/1, eta_ee_ddot_d/1, Integrator1/1
  Gain1/1 -> Sum/1
  Sum/1 -> Gain2/1
  reference/1 -> Scope/1, Gain1/1
  Integrator1/1 -> Integrator/1, Scope1/1, Gain3/1
  Integrator/1 -> To Workspace3/1, Scope3/1, Gain4/1
  Gain3/1 -> Sum/3
  Gain4/1 -> Sum/2
  ? -> To Workspace1/1

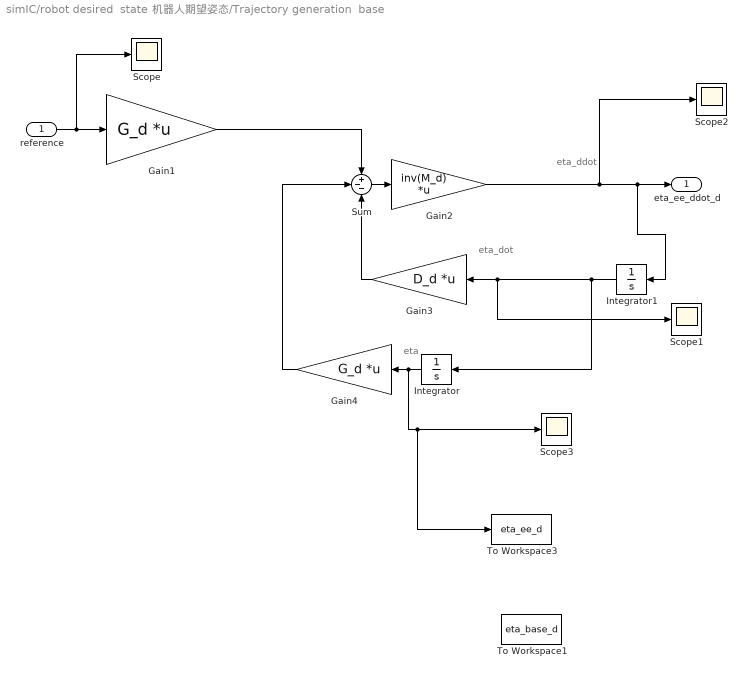
== system simIC/robot desired  state 机器人期望姿态/Trajectory generation  base ==
  note: eta_dot
  note: eta
  note: eta_ddot
  reference : Inport
  Gain1 : Gain  Gain=G_d  Multiplication=Matrix(K*u) (u vector)
  Gain2 : Gain  Gain=inv(M_d)  Multiplication=Matrix(K*u) (u vector)
  Gain3 : Gain  Gain=D_d  Multiplication=Matrix(K*u) (u vector)
  Gain4 : Gain  Gain=G_d  Multiplication=Matrix(K*u) (u vector)
  Integrator : Integrator
  Integrator1 : Integrator
  Scope{,1..3} (4 alike) : Scope
  Sum : Sum  Inputs=+--
  To Workspace1 : ToWorkspace  VariableName=eta_base_d  SaveFormat=Timeseries  SampleTime=-1
  To Workspace3 : ToWorkspace  VariableName=eta_ee_d  SaveFormat=Timeseries  SampleTime=-1
  eta_ee_ddot_d : Outport  VectorParamsAs1DForOutWhenUnconnected=off
  wires:
  Gain2/1 -> Scope2/1, eta_ee_ddot_d/1, Integrator1/1
  Gain1/1 -> Sum/1
  Sum/1 -> Gain2/1
  reference/1 -> Scope/1, Gain1/1
  Integrator1/1 -> Integrator/1, Scope1/1, Gain3/1
  Integrator/1 -> To Workspace3/1, Scope3/1, Gain4/1
  Gain3/1 -> Sum/3
  Gain4/1 -> Sum/2
  ? -> To Workspace1/1

== matlab function simIC/Simulator1/MATLAB Function2 ==
  data: pos_ee_dot output; x input; snake parameter; eta_ee_dot output; omega_ee output; eul_ee_dot output
function [pos_ee_dot,eta_ee_dot, omega_ee,eul_ee_dot] = snake2points(x,snake)

   quat         = x(4:7);
   theta        = x(8 : 6+snake.n);
    zeta      =  x(7+snake.n : 11+2*snake.n);

   
   [R,J]=comp_rot_jac(quat,theta,snake);
   
   eul_ee=rotm2eul(R(:,:,11), 'XYZ')';
   Jinv=Jinv_fromeul(eul_ee);

   eta_ee_dot=[R(:,:,11) zeros(3); zeros(3) Jinv]*J(:,:,11)*zeta;  %%% （2.25）base 位姿速度 在惯性坐标系下
   %% dpos 与 d欧拉角
   pos_ee_dot=eta_ee_dot(1:3);
   eul_ee_dot=eta_ee_dot(4:6);

   x_ee_dot=[R(:,:,11) zeros(3); zeros(3) R(:,:,11)]*J(:,:,11)*zeta;  %%(2.26)
   omega_ee=x_ee_dot(4:6);  %%%(2.26)  在末端执行器的坐标系下
end

== matlab function simIC/Simulator/MATLAB Function2 ==
  data: pos_ee_dot output; x input; snake parameter; eta_ee_dot output; omega_ee output; eul_ee_dot output
function [pos_ee_dot,eta_ee_dot, omega_ee,eul_ee_dot] = snake2points(x,snake)

   quat         = x(4:7);
   theta        = x(8 : 6+snake.n);
    zeta      =  x(7+snake.n : 11+2*snake.n);

   
   [R,J]=comp_rot_jac(quat,theta,snake);
   
   eul_ee=rotm2eul(R(:,:,11), 'XYZ')';
   Jinv=Jinv_fromeul(eul_ee);

   eta_ee_dot=[R(:,:,11) zeros(3); zeros(3) Jinv]*J(:,:,11)*zeta;  %%% （2.25）base 位姿速度 在惯性坐标系下
   %% dpos 与 d欧拉角
   pos_ee_dot=eta_ee_dot(1:3);
   eul_ee_dot=eta_ee_dot(4:6);

   x_ee_dot=[R(:,:,11) zeros(3); zeros(3) R(:,:,11)]*J(:,:,11)*zeta;  %%(2.26)
   omega_ee=x_ee_dot(4:6);  %%%(2.26)  在末端执行器的坐标系下
end

== matlab function simIC/Impedance control1/MATLAB Function4 ==
  data: grip input; eta_ee_des output; eta_ee_ddot_force input; eta_ee_ddot_noforce input
function eta_ee_des = fcn(grip, eta_ee_ddot_force,eta_ee_ddot_noforce)



if grip==1
    eta_ee_des=eta_ee_ddot_force;
else
    eta_ee_des=eta_ee_ddot_noforce;
end

== matlab function simIC/IKinematics1/MATLAB Function1 ==
  data: eta_ee_d_dot input; x input; eta_t_ref input; zeta_ref output; snake parameter; pos_t_ref output; eta_t_dot_quat_ref output; quatt_ref output
function [zeta_ref , pos_t_ref,eta_t_dot_quat_ref, quatt_ref] = fucn(eta_ee_d_dot,x,eta_t_ref, snake)
quat      =  x(4:7);
theta     =  x(8 : 6+snake.n);
[R, J_t]    =  comp_rot_jac(quat,theta,snake);  %%%%  每个关节与base之间的旋转矩阵rot(:,:,i) 雅可比矩阵 jac(:,:,i)   


eul_ee=rotm2eul(R(:,:,11), 'XYZ')';  %%%  旋转矩阵  对应的顺序

Jinv=Jinv_fromeul(eul_ee); %%%%   机器人动力学课程 笔记   （2.88）

J_zuo=[R(:,:,5) zeros(3); zeros(3) Jinv]*J_t(:,:,5);  %（2.25）J_t 体坐标系
J_you=[R(:,:,9) zeros(3); zeros(3) Jinv]*J_t(:,:,9);  %（2.25）J_t 体坐标系

%% (3.4)与（3.2）  加入了权重矩阵W = diag
zeta_ref_zuo=inv(diag([1 1 1 1 1 1 1 1 1 1 1 1 1 1 0.1]))*J_zuo'/(J_zuo*inv(diag([1 1 1 1 1 1 1 1 1 1 1 1 1 1 0.1]))*J_zuo'+0.0001*eye(6))*(eta_zuo_d_dot);    %%%%  关节期望速度
zeta_ref_you=inv(diag([1 1 1 1 1 1 1 1 1 1 1 1 1 1 0.1]))*J'/(J*inv(diag([1 1 1 1 1 1 1 1 1 1 1 1 1 1 0.1]))*J'+0.0001*eye(6))*(eta_you_d_dot);    %%%%  关节期望速度
% 没有权重矩阵  则是（3.3）
% zeta_ref=J'/(J*J'+0.0001*eye(6))*(eta_ee_d_dot);    %%%%  关节期望速度

eta_ee_ref_dot=J*zeta_ref;%(2.25)



quatt_ref=eta_t_ref(4:7);  %%%%   eta_t_ref  为eta_t_dot_quat_ref 的结果积分得到
pos_t_ref=eta_t_ref(1:3);  

R_tail=quat2rotm(quatt_ref');

pos_t_dot   =  R_tail(:,:,1)*zeta_ref(1:3);  %%%%  body（base） 体坐标速度 =  R * V_joint
quat_t_dot  =  TransAngQ(quatt_ref)*zeta_ref(4:6)+1*(1-quatt_ref'*quatt_ref)*quatt_ref; %% T*w + 1*(1-q'*q)*q  %%%(2.19) 公式力的左边表示 实部  虚部  这里的 r 取2  所以变成1 *

eta_t_dot_quat_ref=[pos_t_dot; quat_t_dot];  %3+4 

end

== matlab function simIC/Simulator1/MATLAB Function3 ==
  data: omega_ee input; omega_ee_dot input; pos_ee input; h_ee output size=6; grip input; valve_dot output; valve_pos parameter
function [h_ee,valve_dot]= vent(omega_ee,omega_ee_dot,pos_ee,grip,valve_pos)
x=pos_ee(1);
xe=valve_pos(1);
J_v=3  ;
my_v=500;
if  abs(omega_ee(1))>0 && grip==1
    my_ee=[J_v*omega_ee_dot(1)+my_v*omega_ee(1); 0;0];%%%%  公式2.49   阀门力矩
else
    my_ee=[0 0 0]';
end
f_ee=[0 0 0]';


if (x-xe)>0
    f_ee(1)=20*(x-xe);  %%%2.50
end



h_ee=-[f_ee;my_ee];
%h_ee=[0 0 0 0 0 0]';

if grip==true
    valve_dot=omega_ee(1);
else
    valve_dot=0;
end
end

== matlab function simIC/thrust allocation1/MATLAB Function ==
  data: TCM output; x input; snake parameter
function TCM = fcn(x , snake)
quat      =  x(4:7);
theta     =  x(8 : 6+snake.n);
[~, J]    =  comp_rot_jac(quat,theta,snake);
B        =  comp_TCM(J,snake);


TCM_t=B(1:6,:);

TCM=transpose(TCM_t)/(TCM_t*transpose(TCM_t));%%%%%（3.7）  求的是B^+

== matlab function simIC/IDC 逆动力学/DC/MATLAB Function ==
  data: x input; zeta_dot_r input; reg output; known_input output; snake parameter; pp parameter; gamma parameter; beta parameter; zeta_r input; d output
function [reg, known_input,d] = regressor(x,zeta_dot_r,snake,pp, gamma, beta, zeta_r)

quat      =  x(4:7);
theta     =  x(8 : 6+snake.n);
zeta      =  x(7+snake.n : 11+2*snake.n);
[R, J]    =  comp_rot_jac(quat,theta,snake);
[c,d,g,D] = comp_cdg_adaptiv(J,R,theta,snake,pp,beta,gamma,zeta,zeta_r);
M = comp_mass(J,snake);




drag_matrix=zeros(15,4);
for i=1:snake.n
 drag_matrix=drag_matrix+J(:,:,i)'*D(:,:,i);
end



known_input= M*zeta_dot_r+c+g;  %%%%（4.10） 已知参数部分  为什么不是  M*zeta_dot_r +c*zeta  +g
% known_input= M*zeta_dot_r+  c*zeta  +g;   %%%%修改后

reg=drag_matrix;


end

== matlab function simIC/DC/MATLAB Function4 ==
  data: y_tilde_dot_temp input; eps_tilde_dot input; y_tilde_dot output
function y_tilde_dot = calc_estdot(y_tilde_dot_temp,eps_tilde_dot)

y_tilde_dot=[y_tilde_dot_temp(1:3);eps_tilde_dot;y_tilde_dot_temp(7:15)];
end

== matlab function simIC/IDC 逆动力学/DC/MATLAB Function1 ==
  data: s input; regressor input; estimate_dot output; K_theta parameter
function estimate_dot = calc_estdot(s,regressor,K_theta)


estimate_dot=inv(K_theta)*regressor'*s;  %%%%%(4.11)

end

== matlab function simIC/Simulator/MATLAB Function3 ==
  data: omega_ee input; omega_ee_dot input; pos_ee input; h_ee output size=6; grip input; valve_dot output; valve_pos parameter
function [h_ee,valve_dot]= vent(omega_ee,omega_ee_dot,pos_ee,grip,valve_pos)
x=pos_ee(1);
xe=valve_pos(1);
J_v=3  ;
my_v=500;
if  abs(omega_ee(1))>0 && grip==1
    my_ee=[J_v*omega_ee_dot(1)+my_v*omega_ee(1); 0;0];%%%%  公式2.49   阀门力矩
else
    my_ee=[0 0 0]';
end
f_ee=[0 0 0]';


if (x-xe)>0
    f_ee(1)=20*(x-xe);  %%%2.50
end



h_ee=-[f_ee;my_ee];
%h_ee=[0 0 0 0 0 0]';

if grip==true
    valve_dot=omega_ee(1);
else
    valve_dot=0;
end
end

== matlab function simIC/IDC 逆动力学/DC/MATLAB Function2 ==
  data: x input; estimate input; known_input input; regressor input; u output; s_m input; K_D parameter; snake parameter; d_est output
function [u,d_est]= input(x,estimate,known_input,regressor,s_m, K_D,snake)

quat      =  x(4:7);
theta     =  x(8 : 6+snake.n);

[~, J]    =  comp_rot_jac(quat,theta,snake);


B=comp_TCM(J,snake);
B_u=[eye(6,6) zeros(6,9); B(7:end,:)*pinv(B(1:6,:)) eye(9)];
d_est=regressor*estimate;

u=pinv(B_u)*(K_D*s_m+known_input+regressor*estimate);  %%%%（4.10）   konwn_input 为已知矩阵 M c g


end

== matlab function simIC/IDC 逆动力学/DC/MATLAB Function3 ==
  data: y_tilde input; zeta_tilde input; s_m output; Lambda parameter; K_D parameter; K_P parameter
function s_m = calc_estdot(y_tilde, zeta_tilde, Lambda, K_D, K_P)


s_m=zeta_tilde+Lambda*y_tilde + inv(K_D)*K_P*y_tilde;
end

== matlab function simIC/IDC 逆动力学/DC/MATLAB Function4 ==
  data: y_tilde_dot_temp input; eps_tilde_dot input; y_tilde_dot output
function y_tilde_dot = calc_estdot(y_tilde_dot_temp,eps_tilde_dot)

y_tilde_dot=[y_tilde_dot_temp(1:3);eps_tilde_dot;y_tilde_dot_temp(7:15)];
end

== matlab function simIC/IDC 逆动力学/DC/输出 y_tlide[pos_tilde;quat_tilde; theta_tilde]; 四元数误差虚部 ==
  data: x input; y_tilde output; pos_t_ref input size=3; quat_t_ref input size=4; theta_ref input; eps_tilde_dot output; zeta_ref input
function [y_tilde,eps_tilde_dot] = dyn(x,pos_t_ref, quat_t_ref, theta_ref, zeta_ref)
pos_t=x(1:3);
quat      =  x(4:7);
theta     =  x(8 : 16);
zeta     =  x( 17: 31);

theta_tilde=theta_ref-theta;

pos_tilde=quat2rotm(quat')*(pos_t_ref-pos_t);
pos_tilde2=RotQ(quat)*(pos_t_ref-pos_t);  %%%% 4.12



quat_tilde=quat(1)*quat_t_ref(2:4)-quat_t_ref(1)*quat(2:4)+cross(quat_t_ref(2:4),quat(2:4));%%%虚数部分
eta_tilde = quat(1) * quat_t_ref (1) + quat_t_ref(2:4)'*quat(2:4);%%%%实部  （4.5）

if eta_tilde < 0
quat_tilde = - quat_tilde ;
end


y_tilde=[pos_tilde;quat_tilde; theta_tilde];  %%%4.12

out=pos_t_ref-pos_t;
nu2_tilde=zeta_ref(4:6)-zeta(4:6);%%%%%nu2 ----  V
eps_tilde_dot=0.5*eta_tilde*nu2_tilde + 0.5*skew(quat_tilde)*nu2_tilde;%%%%  四元数误差 虚部=（2.15）
%   skew  求反对称矩阵

end

== matlab function simIC/Simulator/MATLAB Function1 ==
  data: pos_ee input; valve_rotation input; grip output; valve_pos parameter
function grip = vent(pos_ee,valve_rotation,valve_pos)
grip=false;
if abs(pos_ee-valve_pos)<0.3
    grip=true;
%      if valve_rotation(1)>pi/4
%          grip=false;
%      end
end
error=pos_ee-valve_pos;

end

== matlab function simIC/IKinematics2/MATLAB Function1 ==
  data: eta_zuo_d_dot input; eta_you_d_dot input; x input; eta_t_ref input; zeta_ref output; snake parameter; pos_t_ref output; eta_t_dot_quat_ref output; quatt_ref output
function [zeta_ref , pos_t_ref,eta_t_dot_quat_ref, quatt_ref] = fucn(eta_zuo_d_dot,eta_you_d_dot,x,eta_t_ref, snake)
quat      =  x(4:7);
theta     =  x(8 : 6+snake.n);
[R, J_t]    =  comp_rot_jac(quat,theta,snake);  %%%%  每个关节与base之间的旋转矩阵rot(:,:,i) 雅可比矩阵 jac(:,:,i)   


eul_ee=rotm2eul(R(:,:,11), 'XYZ')';  %%%  旋转矩阵  对应的顺序

Jinv=Jinv_fromeul(eul_ee); %%%%   机器人动力学课程 笔记   （2.88）

J_zuo=[R(:,:,5) zeros(3); zeros(3) Jinv]*J_t(:,:,5);  %（2.25）J_t 体坐标系
J_you=[R(:,:,9) zeros(3); zeros(3) Jinv]*J_t(:,:,9);  %（2.25）J_t 体坐标系

%% (3.4)与（3.2）  加入了权重矩阵W = diag
zeta_ref_zuo=inv(diag([1 1 1 1 1 1 1 1 1 1 1 1 1 1 0.1]))*J_zuo'/(J_zuo*inv(diag([1 1 1 1 1 1 1 1 1 1 1 1 1 1 0.1]))*J_zuo'+0.0001*eye(6))*(eta_zuo_d_dot);    %%%%  关节期望速度
zeta_ref_you=inv(diag([1 1 1 1 1 1 1 1 1 1 1 1 1 1 0.1]))*J'/(J*inv(diag([1 1 1 1 1 1 1 1 1 1 1 1 1 1 0.1]))*J'+0.0001*eye(6))*(eta_you_d_dot);    %%%%  关节期望速度
% 没有权重矩阵  则是（3.3）
% zeta_ref=J'/(J*J'+0.0001*eye(6))*(eta_ee_d_dot);    %%%%  关节期望速度

eta_ee_ref_dot=J*zeta_ref;%(2.25)



quatt_ref=eta_t_ref(4:7);  %%%%   eta_t_ref  为eta_t_dot_quat_ref 的结果积分得到

pos_t_ref=eta_t_ref(1:3);  

R_tail=quat2rotm(quatt_ref');

pos_t_dot   =  R_tail(:,:,1)*zeta_ref(1:3);  %%%%  body（base） 体坐标速度 =  R * V_joint
quat_t_dot  =  TransAngQ(quatt_ref)*zeta_ref(4:6)+1*(1-quatt_ref'*quatt_ref)*quatt_ref; %% T*w + 1*(1-q'*q)*q  %%%(2.19) 公式力的左边表示 实部  虚部  这里的 r 取2  所以变成1 *

eta_t_dot_quat_ref=[pos_t_dot; quat_t_dot];  %3+4 

end

== matlab function simIC/DC/MATLAB Function ==
  data: x input; zeta_dot_r input; reg output; known_input output; snake parameter; pp parameter; gamma parameter; beta parameter; zeta_r input; d output
function [reg, known_input,d] = regressor(x,zeta_dot_r,snake,pp, gamma, beta, zeta_r)

quat      =  x(4:7);
theta     =  x(8 : 6+snake.n);
zeta      =  x(7+snake.n : 11+2*snake.n);
[R, J]    =  comp_rot_jac(quat,theta,snake);
[c,d,g,D] = comp_cdg_adaptiv(J,R,theta,snake,pp,beta,gamma,zeta,zeta_r);
M = comp_mass(J,snake);




drag_matrix=zeros(15,4);
for i=1:snake.n
 drag_matrix=drag_matrix+J(:,:,i)'*D(:,:,i);
end



known_input= M*zeta_dot_r+c+g;  %%%%（4.10） 已知参数部分  为什么不是  M*zeta_dot_r +c*zeta  +g
% known_input= M*zeta_dot_r+  c*zeta  +g;   %%%%修改后

reg=drag_matrix;


end

== matlab function simIC/DC/MATLAB Function1 ==
  data: s input; regressor input; estimate_dot output; K_theta parameter
function estimate_dot = calc_estdot(s,regressor,K_theta)


estimate_dot=inv(K_theta)*regressor'*s;  %%%%%(4.11)

end

== matlab function simIC/DC/MATLAB Function2 ==
  data: x input; estimate input; known_input input; regressor input; u output; s_m input; K_D parameter; snake parameter; d_est output
function [u,d_est]= input(x,estimate,known_input,regressor,s_m, K_D,snake)

quat      =  x(4:7);
theta     =  x(8 : 6+snake.n);

[~, J]    =  comp_rot_jac(quat,theta,snake);


B=comp_TCM(J,snake);
B_u=[eye(6,6) zeros(6,9); B(7:end,:)*pinv(B(1:6,:)) eye(9)];
d_est=regressor*estimate;

u=pinv(B_u)*(K_D*s_m+known_input+regressor*estimate);  %%%%（4.10）   konwn_input 为已知矩阵 M c g


end

== matlab function simIC/DC/MATLAB Function3 ==
  data: y_tilde input; zeta_tilde input; s_m output; Lambda parameter; K_D parameter; K_P parameter
function s_m = calc_estdot(y_tilde, zeta_tilde, Lambda, K_D, K_P)


s_m=zeta_tilde+Lambda*y_tilde + inv(K_D)*K_P*y_tilde;
end

== matlab function simIC/DC/输出 y_tlide[pos_tilde;quat_tilde; theta_tilde]; 四元数误差虚部 ==
  data: x input; y_tilde output; pos_t_ref input size=3; quat_t_ref input size=4; theta_ref input; eps_tilde_dot output; zeta_ref input
function [y_tilde,eps_tilde_dot] = dyn(x,pos_t_ref, quat_t_ref, theta_ref, zeta_ref)
pos_t=x(1:3);
quat      =  x(4:7);
theta     =  x(8 : 16);
zeta     =  x( 17: 31);

theta_tilde=theta_ref-theta;

pos_tilde=quat2rotm(quat')*(pos_t_ref-pos_t);
pos_tilde2=RotQ(quat)*(pos_t_ref-pos_t);  %%%% 4.12



quat_tilde=quat(1)*quat_t_ref(2:4)-quat_t_ref(1)*quat(2:4)+cross(quat_t_ref(2:4),quat(2:4));%%%虚数部分
eta_tilde = quat(1) * quat_t_ref (1) + quat_t_ref(2:4)'*quat(2:4);%%%%实部  （4.5）

if eta_tilde < 0
quat_tilde = - quat_tilde ;
end


y_tilde=[pos_tilde;quat_tilde; theta_tilde];  %%%4.12

out=pos_t_ref-pos_t;
nu2_tilde=zeta_ref(4:6)-zeta(4:6);%%%%%nu2 ----  V
eps_tilde_dot=0.5*eta_tilde*nu2_tilde + 0.5*skew(quat_tilde)*nu2_tilde;%%%%  四元数误差 虚部=（2.15）
%   skew  求反对称矩阵

end

== matlab function simIC/Impedance control1/MATLAB Function1 ==
  data: eta_ee_tilde output; eta_ee_d input; eta_ee input
function eta_ee_tilde = fcn(eta_ee_d, eta_ee)

eta_ee1_d=eta_ee_d(1:3);
eta_ee1=eta_ee(1:3);

quat_ee_d=eul2quat(eta_ee_d(4:6)','XYZ')';
quat_ee=eul2quat(eta_ee(4:6)','XYZ')';

quat_error=quat_ee(1)*quat_ee_d(2:4)-quat_ee_d(1)*quat_ee(2:4)-cross(quat_ee_d(2:4),quat_ee(2:4));

eta_ee_tilde=[eta_ee1_d-eta_ee1;quat_error];

== matlab function simIC/Impedance control1/MATLAB Function2 ==
  data: eta_ee_tilde input; eta_ee_des output; eta_ee_tilde_int input; v_tilde input; K_SI parameter; K_DI parameter; K_II parameter
function eta_ee_des = fcn(eta_ee_tilde,eta_ee_tilde_int, v_tilde,K_SI, K_DI, K_II)





eta_ee_force=K_SI*eta_ee_tilde+K_DI*v_tilde+K_II*eta_ee_tilde_int;

%if grip==1
    eta_ee_des=eta_ee_force;
% else
%     eta_ee_des=eta_ee_noforce;
% end

== matlab function simIC/Impedance control1/MATLAB Function3 ==
  data: v_tilde output; eta_ee_dot_d input; eta_ee_dot input; omega_ee input; eta_ee_d input; omega_ee output; omega_ee_d output
function [v_tilde,omega_ee,omega_ee_d] = fcn(eta_ee_dot_d, eta_ee_dot,omega_ee, eta_ee_d)

eta_ee1_dot_d=eta_ee_dot_d(1:3);
eta_ee1_dot=eta_ee_dot(1:3);

eta_ee2_dot_d=eta_ee_dot_d(4:6);


phi=eta_ee_d(4);
theta=eta_ee_d(5);
psi=eta_ee_d(6);

J=[1 0 -sin(theta); 0 cos(theta) cos(theta)*sin(phi); 0 -sin(phi) cos(theta)*cos(phi)];
R=rotx(rad2deg(phi))*roty(rad2deg(theta))*rotz(rad2deg(psi));

omega_ee_d=R*J*eta_ee2_dot_d;
omega_error=omega_ee_d-omega_ee;

v_tilde=[eta_ee1_dot_d-eta_ee1_dot;omega_error];

== matlab function simIC/Simulator1/MATLAB Function ==
  data: x input; x_dot output; joint_torque input; thrust input; grip input; h_ee input; pp parameter; snake parameter; dragcoeff parameter
function x_dot =  MATLAB_Function(x,joint_torque,thrust,grip,h_ee,pp , snake, dragcoeff)

pos       =  x(1:3);
quat      =  x(4:7);
theta     =  x(8 : 6+snake.n);
zeta      =  x(7+snake.n : 11+2*snake.n);  %%%%%（2.20）   = [nu1 ,nu2 , quat_dot ]
%Compute rotation matrices and jacobians
[R, J]    =  comp_rot_jac(quat,theta,snake);
[Rcdg,Jcdg]=comp_rot_jac_mcdg(quat,theta,snake);
%Compute mass matrix
M         =  comp_mass(Jcdg,snake);

%Compute relative velocity to take into account the effect of current 考虑水流影响得到相对加速度
velc_h    =  Rcdg(:,:,1)'*pp.velc;   %水流速度
nu        =  zeta(1:6);
zeta(1:3) =  zeta(1:3)-velc_h;

%Compute coriolis, drag, and hydrostatic terms with the relative velocity
[c, d, g] =  comp_cdg(Jcdg,Rcdg,theta,snake,pp,dragcoeff,zeta);
%Compute the thrust-configuration matrix
B         =  comp_TCM(Jcdg,snake);

%Force
% eul_ee=rotm2eul(R(:,:,11),'XYZ')';
% Jinv=Jinv_fromeul(eul_ee);
% 
% eul_ee_ZYX=rotm2eul(R(:,:,11),'ZYX')';
% eul_ee_ZYZ=rotm2eul(R(:,:,11),'ZYZ')';
% alpha=eul_ee_ZYX(1);
% beta=eul_ee_ZYX(2);
% gamma=eul_ee_ZYX(3);

%Jinv_zyz=inv([cos(eul_ee_ZYZ(2))*sin(eul_ee_ZYZ(3)) -sin(eul_ee_ZYZ(3)) 0; cos(eul_ee_ZYZ(2))*sin(eul_ee_ZYZ(3)) cos(eul_ee_ZYZ(3)) 0; -sin(eul_ee_ZYZ(2)) 0 1]);

%Jinv_zyx=inv([-sin(beta) 0 1;cos(beta)*sin(gamma) cos(gamma) 0; cos(beta)*cos(gamma) -sin(beta) 0]);
%RJ=rotx(rad2deg(eul_ee(1)))*roty(rad2deg(eul_ee(2)))*rotz(rad2deg(eul_ee(3)));
%R(:,:,11);
J_f=[R(:,:,11) zeros(3); zeros(3) R(:,:,11)]*J(:,:,11);



%Compute the relative acceleration
if grip==1
    zeta_dot      =  M\([B [zeros(6,9); eye(9)]]*[thrust;joint_torque]-c-d-g+J_f'*h_ee);
else

    zeta_dot      =  M\([B [zeros(6,9); eye(9)]]*[thrust;joint_torque]-c-d-g);% -c-d-g
end


out=M\[B [zeros(6,9); eye(9)]]*[thrust;joint_torque];
out2=M\(-c-d-g);

%Remove the effect of current  cross 叉积
zeta_dot(1:3) = zeta_dot(1:3)-cross(nu(4:6),velc_h);
%Compute the time derivatives of position and orientation
pos_dot   =  Rcdg(:,:,1)*nu(1:3);  
quat_dot  =  TransAngQ(quat)*nu(4:6)+1*(1-quat'*quat)*quat; 
%Assemble derivative of the state vector
x_dot = [pos_dot ; quat_dot ; zeta(7:snake.n+5) ; zeta_dot];
end

== matlab function simIC/Simulator/MATLAB Function ==
  data: x input; x_dot output; joint_torque input; thrust input; grip input; h_ee input; pp parameter; snake parameter; dragcoeff parameter
function x_dot =  MATLAB_Function(x,joint_torque,thrust,grip,h_ee,pp , snake, dragcoeff)

pos       =  x(1:3);
quat      =  x(4:7);
theta     =  x(8 : 6+snake.n);
zeta      =  x(7+snake.n : 11+2*snake.n);  %%%%%（2.20）   = [nu1 ,nu2 , quat_dot ]
%Compute rotation matrices and jacobians
[R, J]    =  comp_rot_jac(quat,theta,snake);
[Rcdg,Jcdg]=comp_rot_jac_mcdg(quat,theta,snake);
%Compute mass matrix
M         =  comp_mass(Jcdg,snake);

%Compute relative velocity to take into account the effect of current 考虑水流影响得到相对加速度
velc_h    =  Rcdg(:,:,1)'*pp.velc;   %水流速度
nu        =  zeta(1:6);
zeta(1:3) =  zeta(1:3)-velc_h;

%Compute coriolis, drag, and hydrostatic terms with the relative velocity
[c, d, g] =  comp_cdg(Jcdg,Rcdg,theta,snake,pp,dragcoeff,zeta);
%Compute the thrust-configuration matrix
B         =  comp_TCM(Jcdg,snake);

%Force
% eul_ee=rotm2eul(R(:,:,11),'XYZ')';
% Jinv=Jinv_fromeul(eul_ee);
% 
% eul_ee_ZYX=rotm2eul(R(:,:,11),'ZYX')';
% eul_ee_ZYZ=rotm2eul(R(:,:,11),'ZYZ')';
% alpha=eul_ee_ZYX(1);
% beta=eul_ee_ZYX(2);
% gamma=eul_ee_ZYX(3);

%Jinv_zyz=inv([cos(eul_ee_ZYZ(2))*sin(eul_ee_ZYZ(3)) -sin(eul_ee_ZYZ(3)) 0; cos(eul_ee_ZYZ(2))*sin(eul_ee_ZYZ(3)) cos(eul_ee_ZYZ(3)) 0; -sin(eul_ee_ZYZ(2)) 0 1]);

%Jinv_zyx=inv([-sin(beta) 0 1;cos(beta)*sin(gamma) cos(gamma) 0; cos(beta)*cos(gamma) -sin(beta) 0]);
%RJ=rotx(rad2deg(eul_ee(1)))*roty(rad2deg(eul_ee(2)))*rotz(rad2deg(eul_ee(3)));
%R(:,:,11);
J_f=[R(:,:,11) zeros(3); zeros(3) R(:,:,11)]*J(:,:,11);



%Compute the relative acceleration
if grip==1
    zeta_dot      =  M\([B [zeros(6,9); eye(9)]]*[thrust;joint_torque]-c-d-g+J_f'*h_ee);
else

    zeta_dot      =  M\([B [zeros(6,9); eye(9)]]*[thrust;joint_torque]-c-d-g);% -c-d-g
end


out=M\[B [zeros(6,9); eye(9)]]*[thrust;joint_torque];
out2=M\(-c-d-g);

%Remove the effect of current  cross 叉积
zeta_dot(1:3) = zeta_dot(1:3)-cross(nu(4:6),velc_h);
%Compute the time derivatives of position and orientation
pos_dot   =  Rcdg(:,:,1)*nu(1:3);  
quat_dot  =  TransAngQ(quat)*nu(4:6)+1*(1-quat'*quat)*quat; 
%Assemble derivative of the state vector
x_dot = [pos_dot ; quat_dot ; zeta(7:snake.n+5) ; zeta_dot];
end

== matlab function simIC/Simulator1/MATLAB Function1 ==
  data: pos_ee input; valve_rotation input; grip output; valve_pos parameter
function grip = vent(pos_ee,valve_rotation,valve_pos)
grip=false;
if abs(pos_ee-valve_pos)<0.3
    grip=true;
%      if valve_rotation(1)>pi/4
%          grip=false;
%      end
end
error=pos_ee-valve_pos;

end

== matlab function simIC/MATLAB Function ==
  data: t input
function fcn(t)
%#codegen
coder.extrinsic('fprintf');
persistent firstTime

if isempty(firstTime)
    firstTime = false;
    fprintf('Starting Now\n');
end

fprintf('time = %.4f\n',t);

== matlab function simIC/thrust allocation/MATLAB Function ==
  data: TCM output; x input; snake parameter
function TCM = fcn(x , snake)
quat      =  x(4:7);
theta     =  x(8 : 6+snake.n);
[~, J]    =  comp_rot_jac(quat,theta,snake);
B        =  comp_TCM(J,snake);


TCM_t=B(1:6,:);

TCM=transpose(TCM_t)/(TCM_t*transpose(TCM_t));%%%%%（3.7）  求的是B^+
